simulink model "fir_dbl_tap_test"  (Simulink 7.2)
settings: Solver=VariableStepDiscrete  StartTime=0.0  StopTime=50  RelTol=1e-3
libraries: xbsIndex_r4 x18
settings Model: Creator=User  LastModifiedBy=root
settings OptimizationCC: InitFltsAndDblsToZero=on
settings DebuggingCC: SaveWithDisabledLinksMsg=none  SaveWithParameterizedLinksMsg=none

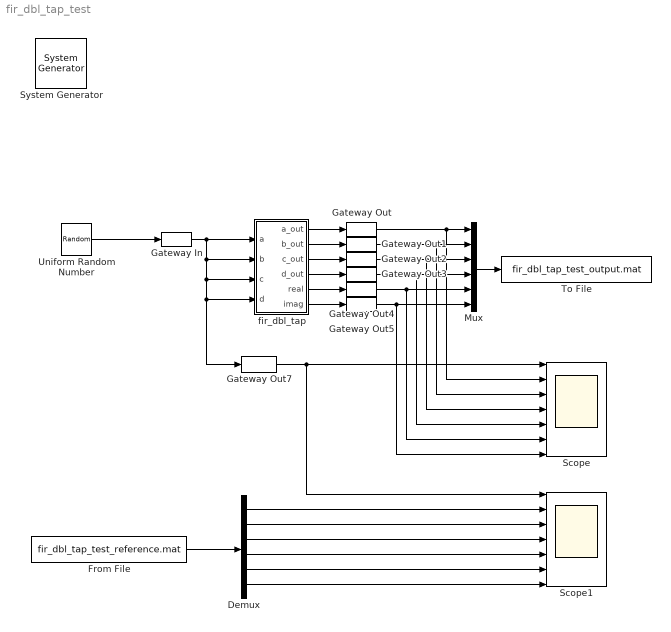
== system fir_dbl_tap_test ==
  " System Generator" : xbsIndex_r4/ System Generator  Tag=genX  SystemSampleTime=-1  xilinxfamily=Virtex4  part=xc4vsx35  speed=-10  package=ff668  synthesis_tool=XST  clock_wrapper=Clock Enables  directory=./netlist  testbench=off  simulink_period=1  sysclk_period=100  dcm_input_clock_period=100  incr_netlist=off  trim_vbits=Everywhere in SubSystem  dbl_ovrd=According to Block Masks  core_generation=According to Block Masks  run_coregen=off  deprecated_control=off  eval_field=0  block_type=sysgen
      settings: block_version=10.1.1
  Demux : Demux  Outputs=6
  From File : FromFile  FileName=fir_dbl_tap_test_reference.mat  SampleTime=1
  Gateway In : xbsIndex_r4/Gateway In  arith_type="Signed  (2's comp)"  n_bits=16  bin_pt=15  quantization=Truncate  overflow=Wrap  period=1  dbl_ovrd=off  timing_constraint=None  locs_specified=off  LOCs={}  hdl_port=on  block_type=gatewayin
      settings: infoedit="Gateway in block.  Converts inputs of type Simulink integer, double and fixed point to  Xilinx fixed point type.<P><P>Hardware notes:  In hardware these blocks become top level input ports."  block_version=10.1.1
  Gateway Out{,1..5,7} (7 alike) : xbsIndex_r4/Gateway Out  hdl_port=on  timing_constraint=None  locs_specified=off  LOCs={}  block_type=gatewayout
      Gateway Out settings: infoedit="Gateway out block.  Converts Xilinx fixed point inputs into ouputs of type Simulink integer, double, or fixed point.<P><P>Hardware notes:  In hardware these blocks become top level output ports or are discarded, depending on how they are configured."  block_version=10.1.1
      Gateway Out1 settings: infoedit="Gateway out block.  Converts Xilinx fixed point inputs into ouputs of type Simulink integer, double, or fixed point.<P><P>Hardware notes:  In hardware these blocks become top level output ports or are discarded, depending on how they are configured."  block_version=10.1.1
      Gateway Out2 settings: infoedit="Gateway out block.  Converts Xilinx fixed point inputs into ouputs of type Simulink integer, double, or fixed point.<P><P>Hardware notes:  In hardware these blocks become top level output ports or are discarded, depending on how they are configured."  block_version=10.1.1
      Gateway Out3 settings: infoedit="Gateway out block.  Converts Xilinx fixed point inputs into ouputs of type Simulink integer, double, or fixed point.<P><P>Hardware notes:  In hardware these blocks become top level output ports or are discarded, depending on how they are configured."  block_version=10.1.1
      Gateway Out4 settings: infoedit="Gateway out block.  Converts Xilinx fixed point inputs into ouputs of type Simulink integer, double, or fixed point.<P><P>Hardware notes:  In hardware these blocks become top level output ports or are discarded, depending on how they are configured."  block_version=10.1.1
      Gateway Out5 settings: infoedit="Gateway out block.  Converts Xilinx fixed point inputs into ouputs of type Simulink integer, double, or fixed point.<P><P>Hardware notes:  In hardware these blocks become top level output ports or are discarded, depending on how they are configured."  block_version=10.1.1
      Gateway Out7 settings: infoedit="Gateway out block.  Converts Xilinx fixed point inputs into ouputs of type Simulink integer, double, or fixed point.<br><br>Hardware notes:  In hardware these blocks become top level output ports or are discarded, depending on how they are configured."  block_version=11.4
  Mux : Mux  Inputs=6
  Scope : Scope  NumInputPorts=7
      settings: YMin=-5~-5~-5~-5~-5~-5~-5  YMax=5~5~5~5~5~5~5
  Scope1 : Scope  NumInputPorts=7
      settings: YMin=-5~-5~-5~-5~-5~-5~-5  YMax=5~5~5~5~5~5~5
  To File : ToFile  Filename=fir_dbl_tap_test_output.mat  MatrixName=output
  Uniform Random Number : UniformRandomNumber  SampleTime=1
  fir_dbl_tap : Subsystem  mask(fir_dbl_tap){factor=0.1234, add_latency=3, mult_latency=4, coeff_bit_width=18, coeff_bin_pt=17}
      mask prompts: add_latency "Add latency"; mult_latency "Mult latency"; coeff_bit_width "Coefficient bit width"; coeff_bin_pt "Coefficient binary point"
      mask Help: eval('xlWeb(''http://casper.berkeley.edu/wiki/Fir_dbl_tap'')')
  wires:
  Uniform Random Number/1 -> Gateway In/1
  Gateway In/1 -> fir_dbl_tap/1(a), fir_dbl_tap/2(b), fir_dbl_tap/3(c), fir_dbl_tap/4(d), Gateway Out7/1
  fir_dbl_tap/1(a_out) -> Gateway Out/1
  fir_dbl_tap/2(b_out) -> Gateway Out1/1
  fir_dbl_tap/3(c_out) -> Gateway Out2/1
  fir_dbl_tap/4(d_out) -> Gateway Out3/1
  fir_dbl_tap/5(real) -> Gateway Out4/1
  fir_dbl_tap/6(imag) -> Gateway Out5/1
  Gateway Out/1 -> Mux/1, Scope/2
  Gateway Out1/1 -> Mux/2, Scope/3
  Gateway Out2/1 -> Mux/3, Scope/4
  Gateway Out3/1 -> Mux/4, Scope/5
  Gateway Out4/1 -> Mux/5, Scope/6
  Gateway Out5/1 -> Mux/6, Scope/7
  Mux/1 -> To File/1
  From File/1 -> Demux/1
  Demux/1 -> Scope1/2
  Demux/2 -> Scope1/3
  Demux/3 -> Scope1/4
  Demux/4 -> Scope1/5
  Demux/5 -> Scope1/6
  Demux/6 -> Scope1/7
  Gateway Out7/1 -> Scope1/1, Scope/1

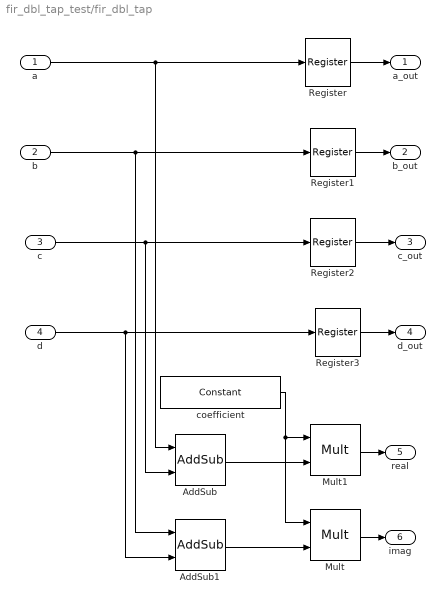
== system fir_dbl_tap_test/fir_dbl_tap ==
  a : Inport  OutDataType=sfix(16)  OutScaling=2^0
  b : Inport  Port=2  OutDataType=sfix(16)  OutScaling=2^0
  c : Inport  Port=3  OutDataType=sfix(16)  OutScaling=2^0
  d : Inport  Port=4  OutDataType=sfix(16)  OutScaling=2^0
  AddSub : xbsIndex_r4/AddSub  mode=Addition  use_carryin=off  use_carryout=off  en=off  latency=add_latency  precision=Full  arith_type="Signed  (2's comp)"  n_bits=18  bin_pt=16  quantization=Truncate  overflow=Wrap  dbl_ovrd=off  use_behavioral_HDL=on  hw_selection=Fabric  pipelined=off  use_rpm=on  block_type=addsub
      settings: xl_area=[0, 0, 0, 0, 0, 0, 0]  block_version=9.2.01
  AddSub1 : xbsIndex_r4/AddSub  mode=Addition  use_carryin=off  use_carryout=off  en=off  latency=add_latency  precision=Full  arith_type="Signed  (2's comp)"  n_bits=18  bin_pt=16  quantization=Truncate  overflow=Wrap  dbl_ovrd=off  use_behavioral_HDL=on  hw_selection=Fabric  pipelined=off  use_rpm=on  block_type=addsub
      settings: xl_area=[0, 0, 0, 0, 0, 0, 0]  block_version=9.2.01
  Mult : xbsIndex_r4/Mult  precision=Full  arith_type="Signed  (2's comp)"  n_bits=18  bin_pt=17  quantization=Truncate  overflow=Wrap  en=off  latency=mult_latency  dbl_ovrd=off  use_behavioral_HDL=on  opt=Speed  use_embedded=on  optimum_pipeline=off  pipeline=on  use_rpm=off  placement_style=Rectangular shape  block_type=mult
      settings: infoedit=Hardware notes: To use the internal pipeline stage of the dedicated multiplier you must select 'Pipeline for maximum performance'.  xl_area=[0, 0, 0, 0, 0, 0, 0]  block_version=9.2.01
  Mult1 : xbsIndex_r4/Mult  precision=Full  arith_type="Signed  (2's comp)"  n_bits=18  bin_pt=17  quantization=Truncate  overflow=Wrap  en=off  latency=mult_latency  dbl_ovrd=off  use_behavioral_HDL=on  opt=Speed  use_embedded=on  optimum_pipeline=off  pipeline=on  use_rpm=off  placement_style=Rectangular shape  block_type=mult
      settings: infoedit=Hardware notes: To use the internal pipeline stage of the dedicated multiplier you must select 'Pipeline for maximum performance'.  xl_area=[0, 0, 0, 0, 0, 0, 0]  block_version=9.2.01
  Register{,1..3} (4 alike) : xbsIndex_r4/Register  init=0  rst=off  en=off  dbl_ovrd=off  block_type=register
      settings: xl_area=[0, 0, 0, 0, 0, 0, 0]  block_version=9.2.01
  coefficient : xbsIndex_r4/Constant  arith_type=Signed (2's comp)  const=factor  n_bits=coeff_bit_width  bin_pt=coeff_bin_pt  explicit_period=on  period=1  equ=P=C  opselect=C  inp2=PCIN>>17  opr=+  inp1=P  carry=CIN  dbl_ovrd=off  block_type=constant
      settings: block_version=9.2.01
  a_out : Outport  OutDataType=sfix(16)  OutScaling=2^0
  b_out : Outport  Port=2  OutDataType=sfix(16)  OutScaling=2^0
  c_out : Outport  Port=3  OutDataType=sfix(16)  OutScaling=2^0
  d_out : Outport  Port=4  OutDataType=sfix(16)  OutScaling=2^0
  real : Outport  Port=5  OutDataType=sfix(16)  OutScaling=2^0
  imag : Outport  Port=6  OutDataType=sfix(16)  OutScaling=2^0
  wires:
  Register1/1 -> b_out/1
  Register/1 -> a_out/1
  coefficient/1 -> Mult/1, Mult1/1
  Mult/1 -> imag/1
  Mult1/1 -> real/1
  Register3/1 -> d_out/1
  Register2/1 -> c_out/1
  a/1 -> Register/1, AddSub/1
  b/1 -> Register1/1, AddSub1/1
  c/1 -> Register2/1, AddSub/2
  d/1 -> Register3/1, AddSub1/2
  AddSub/1 -> Mult1/2
  AddSub1/1 -> Mult/2
